simulink subsystem "ACTUATORS"  (R2025b)
settings: Solver=VariableStepAuto  StartTime=0.0  StopTime=10.0  RelTol=1e-3
undefined symbols (not defined in the file): simData
settings Model: Creator=antoniohernandez-rodiciomateos  LastModifiedBy=antoniohernandez-rodiciomateos

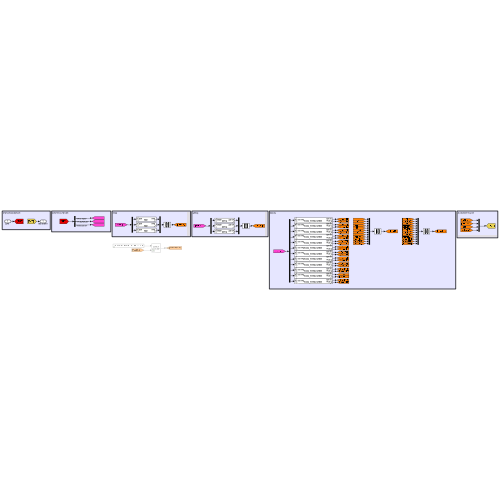
[thumbnail: Simulink's stored preview of the top-level diagram]
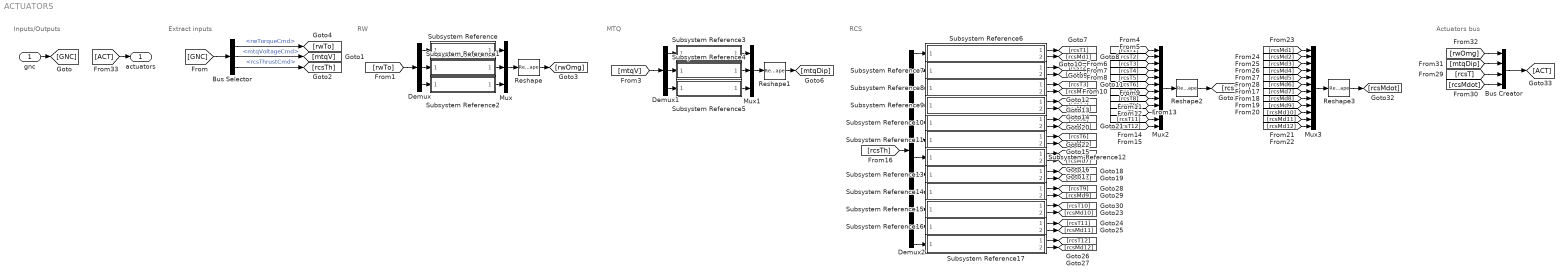
== system ACTUATORS ==
  note: Inputs/Outputs
  note: Extract inputs
  note: RW
  note: MTQ
  note: RCS
  note: Actuators bus
  gnc : Inport  OutDataTypeStr=Bus: gnc_bus
  Bus Creator : BusCreator  Inputs=4  OutDataTypeStr=Bus: actuators_bus  NonVirtualBus=on
      settings: InheritFromInputs=off
  Bus Selector : BusSelector  OutputSignals=rwTorqueCmd,mtqVoltageCmd,rcsThrustCmd
  Demux : Demux  Outputs=3
  Demux1 : Demux  Outputs=3
  Demux2 : Demux  Outputs=12
  Mux : Mux  Inputs=3
  Mux1 : Mux  Inputs=3
  Mux2 : Mux  Inputs=12
  Mux3 : Mux  Inputs=12
  Reshape{,1..3} (4 alike) : Reshape  OutputDimensionality=Column vector (2-D)
  Subsystem Reference : Subsystem  ReferencedSubsystem=RW  rwInertia=simData.rw.rwInertia(1)  rwMaxOmg=simData.rw.rwMaxOmg(1)  rwInitOmg=simData.ic.rwInitOmg(1)
  Subsystem Reference1 : Subsystem  ReferencedSubsystem=RW  rwInertia=simData.rw.rwInertia(2)  rwMaxOmg=simData.rw.rwMaxOmg(2)  rwInitOmg=simData.ic.rwInitOmg(2)
  Subsystem Reference10 : Subsystem  ReferencedSubsystem=RCS_THRUSTER  rcsIsp=simData.rcs.rcsIsp(5)  rcsMaxMdot=simData.rcs.rcsMaxMdot(5)
  Subsystem Reference11 : Subsystem  ReferencedSubsystem=RCS_THRUSTER  rcsIsp=simData.rcs.rcsIsp(6)  rcsMaxMdot=simData.rcs.rcsMaxMdot(6)
  Subsystem Reference12 : Subsystem  ReferencedSubsystem=RCS_THRUSTER  rcsIsp=simData.rcs.rcsIsp(7)  rcsMaxMdot=simData.rcs.rcsMaxMdot(7)
  Subsystem Reference13 : Subsystem  ReferencedSubsystem=RCS_THRUSTER  rcsIsp=simData.rcs.rcsIsp(8)  rcsMaxMdot=simData.rcs.rcsMaxMdot(8)
  Subsystem Reference14 : Subsystem  ReferencedSubsystem=RCS_THRUSTER  rcsIsp=simData.rcs.rcsIsp(9)  rcsMaxMdot=simData.rcs.rcsMaxMdot(9)
  Subsystem Reference15 : Subsystem  ReferencedSubsystem=RCS_THRUSTER  rcsIsp=simData.rcs.rcsIsp(10)  rcsMaxMdot=simData.rcs.rcsMaxMdot(10)
  Subsystem Reference16 : Subsystem  ReferencedSubsystem=RCS_THRUSTER  rcsIsp=simData.rcs.rcsIsp(11)  rcsMaxMdot=simData.rcs.rcsMaxMdot(11)
  Subsystem Reference17 : Subsystem  ReferencedSubsystem=RCS_THRUSTER  rcsIsp=simData.rcs.rcsIsp(12)  rcsMaxMdot=simData.rcs.rcsMaxMdot(12)
  Subsystem Reference2 : Subsystem  ReferencedSubsystem=RW  rwInertia=simData.rw.rwInertia(3)  rwMaxOmg=simData.rw.rwMaxOmg(3)  rwInitOmg=simData.ic.rwInitOmg(3)
  Subsystem Reference3 : Subsystem  ReferencedSubsystem=MTQ  mtqMagneticGain=simData.mtq.mtqMagneticGain(1)  mtqResistance=simData.mtq.mtqResistance(1)  mtqMaxVoltage=simData.mtq.mtqMaxVoltage(1)
  Subsystem Reference4 : Subsystem  ReferencedSubsystem=MTQ  mtqMagneticGain=simData.mtq.mtqMagneticGain(2)  mtqResistance=simData.mtq.mtqResistance(2)  mtqMaxVoltage=simData.mtq.mtqMaxVoltage(2)
  Subsystem Reference5 : Subsystem  ReferencedSubsystem=MTQ  mtqMagneticGain=simData.mtq.mtqMagneticGain(3)  mtqResistance=simData.mtq.mtqResistance(3)  mtqMaxVoltage=simData.mtq.mtqMaxVoltage(3)
  Subsystem Reference6 : Subsystem  ReferencedSubsystem=RCS_THRUSTER  rcsIsp=simData.rcs.rcsIsp(1)  rcsMaxMdot=simData.rcs.rcsMaxMdot(1)
  Subsystem Reference7 : Subsystem  ReferencedSubsystem=RCS_THRUSTER  rcsIsp=simData.rcs.rcsIsp(2)  rcsMaxMdot=simData.rcs.rcsMaxMdot(2)
  Subsystem Reference8 : Subsystem  ReferencedSubsystem=RCS_THRUSTER  rcsIsp=simData.rcs.rcsIsp(3)  rcsMaxMdot=simData.rcs.rcsMaxMdot(3)
  Subsystem Reference9 : Subsystem  ReferencedSubsystem=RCS_THRUSTER  rcsIsp=simData.rcs.rcsIsp(4)  rcsMaxMdot=simData.rcs.rcsMaxMdot(4)
  actuators : Outport  OutDataTypeStr=Bus: actuators_bus
  wires:
  gnc/1 -> [GNC]
  [GNC] -> Bus Selector/1
  [rwTo] -> Demux/1
  Demux/1 -> Subsystem Reference/1
  Demux/2 -> Subsystem Reference1/1
  Demux/3 -> Subsystem Reference2/1
  Subsystem Reference1/1 -> Mux/2
  Subsystem Reference/1 -> Mux/1
  Subsystem Reference2/1 -> Mux/3
  Mux/1 -> Reshape/1
  Reshape/1 -> [rwOmg]
  [mtqV] -> Demux1/1
  Subsystem Reference4/1 -> Mux1/2
  Mux1/1 -> Reshape1/1
  Demux1/2 -> Subsystem Reference4/1
  Demux1/1 -> Subsystem Reference3/1
  Subsystem Reference3/1 -> Mux1/1
  Demux1/3 -> Subsystem Reference5/1
  Subsystem Reference5/1 -> Mux1/3
  Reshape1/1 -> [mtqDip]
  Demux2/1 -> Subsystem Reference6/1
  Demux2/2 -> Subsystem Reference7/1
  Demux2/3 -> Subsystem Reference8/1
  Demux2/4 -> Subsystem Reference9/1
  Demux2/5 -> Subsystem Reference10/1
  Demux2/9 -> Subsystem Reference14/1
  Demux2/10 -> Subsystem Reference15/1
  Demux2/11 -> Subsystem Reference16/1
  Demux2/12 -> Subsystem Reference17/1
  Demux2/8 -> Subsystem Reference13/1
  Demux2/6 -> Subsystem Reference11/1
  Demux2/7 -> Subsystem Reference12/1
  Subsystem Reference6/1 -> [rcsT1]
  Subsystem Reference6/2 -> [rcsMd1]
  Subsystem Reference7/1 -> [rcsT2]
  Subsystem Reference7/2 -> [rcsMd2]
  Subsystem Reference8/1 -> [rcsT3]
  Subsystem Reference8/2 -> [rcsMd3]
  Subsystem Reference9/1 -> [rcsT4]
  Subsystem Reference9/2 -> [rcsMd4]
  Subsystem Reference10/1 -> [rcsT5]
  Subsystem Reference10/2 -> [rcsMd5]
  Subsystem Reference11/1 -> [rcsT6]
  Subsystem Reference11/2 -> [rcsMd6]
  Subsystem Reference12/1 -> [rcsT7]
  Subsystem Reference12/2 -> [rcsMd7]
  Subsystem Reference13/1 -> [rcsT8]
  Subsystem Reference13/2 -> [rcsMd8]
  Subsystem Reference14/1 -> [rcsT9]
  Subsystem Reference14/2 -> [rcsMd9]
  Subsystem Reference15/1 -> [rcsT10]
  Subsystem Reference15/2 -> [rcsMd10]
  Subsystem Reference16/1 -> [rcsT11]
  Subsystem Reference16/2 -> [rcsMd11]
  Subsystem Reference17/1 -> [rcsT12]
  Subsystem Reference17/2 -> [rcsMd12]
  [rcsT1] -> Mux2/1
  [rcsT2] -> Mux2/2
  [rcsT3] -> Mux2/3
  [rcsT4] -> Mux2/4
  [rcsT5] -> Mux2/5
  [rcsT6] -> Mux2/6
  [rcsT7] -> Mux2/7
  [rcsT8] -> Mux2/8
  [rcsT9] -> Mux2/9
  [rcsT10] -> Mux2/10
  [rcsT11] -> Mux2/11
  [rcsT12] -> Mux2/12
  Mux2/1 -> Reshape2/1
  [rcsTh] -> Demux2/1
  Reshape2/1 -> [rcsT]
  [rcsMd3] -> Mux3/3
  [rcsMd6] -> Mux3/6
  [rcsMd8] -> Mux3/8
  [rcsMd12] -> Mux3/12
  [rcsMd2] -> Mux3/2
  [rcsMd5] -> Mux3/5
  [rcsMd9] -> Mux3/9
  Mux3/1 -> Reshape3/1
  [rcsMd11] -> Mux3/11
  [rcsMd1] -> Mux3/1
  Reshape3/1 -> [rcsMdot]
  [rcsMd10] -> Mux3/10
  [rcsMd4] -> Mux3/4
  [rcsMd7] -> Mux3/7
  [rwOmg] -> Bus Creator/1
  [mtqDip] -> Bus Creator/2
  [rcsT] -> Bus Creator/3
  [rcsMdot] -> Bus Creator/4
  [ACT] -> actuators/1
  Bus Creator/1 -> [ACT]
  Bus Selector/1 -> [rwTo]  "<rwTorqueCmd>"
  Bus Selector/2 -> [mtqV]  "<mtqVoltageCmd>"
  Bus Selector/3 -> [rcsTh]  "<rcsThrustCmd>"
